simulink model "SoftwareSystem"  (R2016a)
settings: Solver=FixedStepAuto  StartTime=0.0  StopTime=10.0  FixedStep=0.1  RelTol=1e-3
settings Model: Creator=Josef  LastModifiedBy=Josef
settings GRTTargetCC: GeneratePreprocessorConditionals=Use local settings

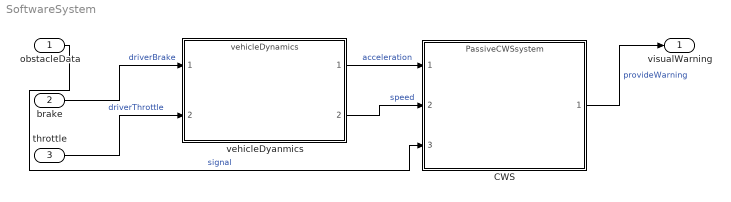
== system SoftwareSystem ==
  obstacleData : Inport
      settings: AttributesFormatString=signal
  brake : Inport  Port=2
      settings: AttributesFormatString=driverBrake
  throttle : Inport  Port=3
      settings: AttributesFormatString=driverThrottle
  CWS : ModelReference  ModelNameDialog=PassiveCWSsystem  SimulationMode=Normal  ModelReferenceVersion=1.16
  vehicleDyanmics : ModelReference  ModelNameDialog=vehicleDynamics  SimulationMode=Normal  ModelReferenceVersion=1.8
  visualWarning : Outport
      settings: AttributesFormatString=provideWarning
  wires:
  vehicleDyanmics/1 -> CWS/1  "acceleration"
  vehicleDyanmics/2 -> CWS/2  "speed"
  CWS/1 -> visualWarning/1  "provideWarning"
  brake/1 -> vehicleDyanmics/1  "driverBrake"
  throttle/1 -> vehicleDyanmics/2  "driverThrottle"
  obstacleData/1 -> CWS/3  "signal"
